simulink model "lab2_sin"  (Simulink 7.9)
settings: Solver=ode45  StartTime=0.0  StopTime=2.0  RelTol=1e-3
settings Model: Creator=Aquirel  LastModifiedBy=Aquirel

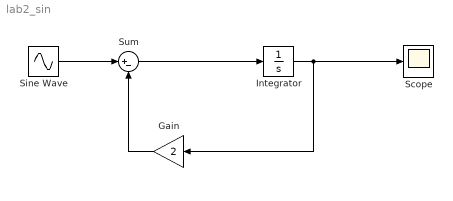
== system lab2_sin ==
  Gain : Gain  Gain=2
  Integrator : Integrator
  Scope : Scope
  Sine Wave : Sin  SampleTime=0
  Sum : Sum  Inputs=|+-
  wires:
  Sine Wave/1 -> Sum/1
  Gain/1 -> Sum/2
  Sum/1 -> Integrator/1
  Integrator/1 -> Gain/1, Scope/1
